simulink model "Hardware_Diagnostics_Test_backup"  (R2025b)
settings: Solver=FixedStepDiscrete  StartTime=0.0  StopTime=inf  FixedStep=0.001  RelTol=1e-3  EnableMultiTasking=on
undefined symbols (not defined in the file or in its folder): bit, Down, GPTRIP1SEL, GPTRIP2SEL, TZ1, TZ2, Up
libraries: c2802xlib x5, c280xlib x3, c2806xlib x2

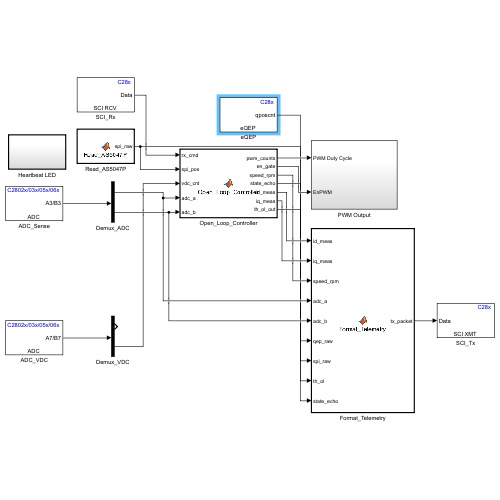
[thumbnail: Simulink's stored preview of the top-level diagram]
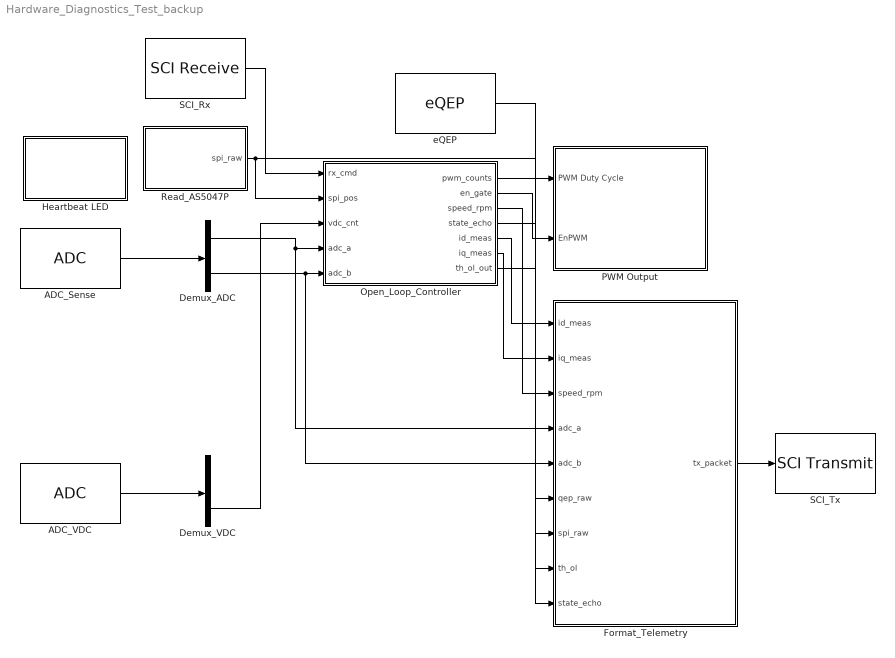
== system Hardware_Diagnostics_Test_backup ==
  ADC_Sense : c2802xlib/ADC  blkParamProc=C2000  ADCModule=1  samplingMode=Simultaneous sample mode  ADCResolution=12-bit (Single-ended input)  ADC29xResolution=12-bit  ADCMode=Single-ended input  useSOC1=SOC0  useSOC2=SOC0_SOC1  SOCAcquisitionWindow=7  SOCTriggerSource=Software  SOCInterruptTrigger=No ADCINT  Ts=-1  dType=uint16  postInterrupt=on  interruptSel=ADCINT1  ADCINTContinuous=on  endma=off  chdma=1  conv1=ADCINA0  conv2=ADCINA3 and ADCINB3  conv1_Type4=ADCIN0  conv2_Type4=ADCIN0 and ADCIN1
  ADC_VDC : c2802xlib/ADC  blkParamProc=C2000  ADCModule=1  samplingMode=Simultaneous sample mode  ADCResolution=12-bit (Single-ended input)  ADC29xResolution=12-bit  ADCMode=Single-ended input  useSOC1=SOC2  useSOC2=SOC2_SOC3  SOCAcquisitionWindow=7  SOCTriggerSource=Software  SOCInterruptTrigger=No ADCINT  Ts=-1  dType=uint16  postInterrupt=off  interruptSel=ADCINT1  ADCINTContinuous=on  endma=off  chdma=1  conv1=ADCINB7  conv2=ADCINA7 and ADCINB7  conv1_Type4=ADCIN0  conv2_Type4=ADCIN0 and ADCIN1
  Demux_ADC : Demux  Outputs=2
  Demux_VDC : Demux  Outputs=2
  Format_Telemetry : MATLAB Function  TreatAsAtomicUnit=on
  Heartbeat LED : Subsystem  TreatAsAtomicUnit=on
  Open_Loop_Controller : MATLAB Function  TreatAsAtomicUnit=on
  PWM Output : Subsystem
  Read_AS5047P : MATLAB Function  TreatAsAtomicUnit=on
  SCI_Rx : c280xlib/SCI Receive  Priority=2  sciModule=A  dataHead=''  headerCheckMaxCount=16  dataTail=''  dataType=uint8  dataLenOptions=Length via dialog  dataDim=1  maxDataLength=1  initValue=0  errOption=Output the last received value  errValue=0  sampleTime=0.001  blockingMode=off  timeOut=inf  outputStatus=off
  SCI_Tx : c280xlib/SCI Transmit  sciModule=A  dataHead='S'  dataTail='E'  frameSize=1  blockingMode=on  outputStatus=off
  eQEP : c280xlib/eQEP  useModule=eQEP1  pcInputmode=Quadrature-count  externalClockrate=2x resolution: Count the rising/falling edge  swapPolarityselection=Clockwise  qdfOutputport=off  qapPolarityselection=off  qbpPolarityselection=off  qipPolarityselection=off  qspPolarityselection=off  igatePolarityselection=off  sampleTime=0.001  pcOutputport=on  pcMaximumvalue=4095  indexInitializationcheck=off  indexInitializationevent=Falling edge  strobeInitializationcheck=off  strobeInitializationevent=Rising edge  softwareInitializationcheck=off  softwareInitializationsource=Set to init value at start up  softwareInitializationmode=on  pcInitialvalue=0  pcResetmode=Reset on the maximum position  ieloutputport=off  indexEventlatch=Rising edge  seloutputport=off  strobeEventlatch=Rising edge  pcefOutputport=off  enableEqepcapture=off  qctmrOutputport=off  qcprdOutputport=off  captureTimerprescaler=128  upEventprescaler=128  overflowErrorflag=off  directionErrorflag=off  captureTimerposition=On position counter read  unitTimerperiod=100000000  captureTimerlatch=off  capturePeriodlatch=off  positionCounterlatch=off  soenPolarityselection=off  spselPolarityselection=Index pin is used for sync output  compareValuesource=Specify via dialog  shadowMode=Load on QPOSCNT=0  compareValue=4294967295  syncOutputwidth=1  polaritySyncoutput=Active high  watchdogEnable=off  watchdogTimer=65535  outport1Datatype=auto  outport2Datatype=auto  outport3Datatype=auto  outport4Datatype=auto  outport5Datatype=auto  outport6Datatype=auto  outport7Datatype=auto  outport8Datatype=auto  outport9Datatype=auto  outport10Datatype=auto  outport11Datatype=auto  outport12Datatype=auto  eqepinterrupt_pce=off  eqepinterrupt_qpe=off  eqepinterrupt_qdc=off  eqepinterrupt_wto=off  eqepinterrupt_pcu=off  eqepinterrupt_pco=off  eqepinterrupt_pcr=off  eqepinterrupt_pcm=off  eqepinterrupt_sel=off  eqepinterrupt_iel=off  eqepinterrupt_uto=off  pheOutputport=off  watchdogOutputport=off  outport13Datatype=auto  outport14Datatype=auto
  wires:
  SCI_Rx/1 -> Open_Loop_Controller/1(rx_cmd)
  ADC_Sense/1 -> Demux_ADC/1
  Demux_ADC/2 -> Open_Loop_Controller/5(adc_b), Format_Telemetry/5(adc_b)
  Read_AS5047P/1(spi_raw) -> Open_Loop_Controller/2(spi_pos), Format_Telemetry/7(spi_raw)
  ADC_VDC/1 -> Demux_VDC/1
  Demux_ADC/1 -> Open_Loop_Controller/4(adc_a), Format_Telemetry/4(adc_a)
  Open_Loop_Controller/1(pwm_counts) -> PWM Output/1(PWM Duty Cycle)
  Open_Loop_Controller/2(en_gate) -> PWM Output/2(EnPWM)
  Format_Telemetry/1(tx_packet) -> SCI_Tx/1
  Open_Loop_Controller/5(id_meas) -> Format_Telemetry/1(id_meas)
  Open_Loop_Controller/6(iq_meas) -> Format_Telemetry/2(iq_meas)
  Open_Loop_Controller/3(speed_rpm) -> Format_Telemetry/3(speed_rpm)
  Demux_VDC/2 -> Open_Loop_Controller/3(vdc_cnt)
  eQEP/1 -> Format_Telemetry/6(qep_raw)
  Open_Loop_Controller/7(th_ol_out) -> Format_Telemetry/8(th_ol)
  Open_Loop_Controller/4(state_echo) -> Format_Telemetry/9(state_echo)

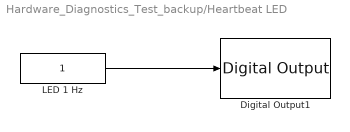
== system Hardware_Diagnostics_Test_backup/Heartbeat LED ==
  Digital Output1 : c2806xlib/Digital Output  GPIO_Number=GPIO32~GPIO39  GPIO_Bit0=off  GPIO_BIT0_Toggle=off  GPIO_Bit1=off  GPIO_BIT1_Toggle=off  GPIO_Bit2=on  GPIO_BIT2_Toggle=on  GPIO_Bit3=off  GPIO_BIT3_Toggle=off  GPIO_Bit4=off  GPIO_BIT4_Toggle=off  GPIO_Bit5=off  GPIO_BIT5_Toggle=off  GPIO_Bit6=off  GPIO_BIT6_Toggle=off  GPIO_Bit7=off  GPIO_BIT7_Toggle=off
  LED 1 Hz : Constant  OutDataTypeStr=uint16  SampleTime=0.5
  wires:
  LED 1 Hz/1 -> Digital Output1/1

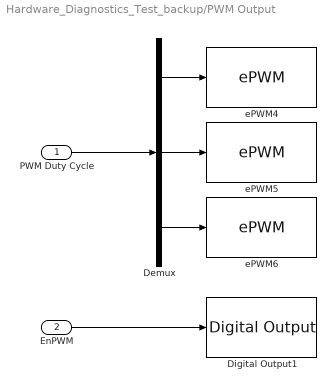
== system Hardware_Diagnostics_Test_backup/PWM Output ==
  PWM Duty Cycle : Inport
  EnPWM : Inport  Port=2
  Demux : Demux  Outputs=3
  Digital Output1 : c2806xlib/Digital Output  GPIO_Number=GPIO50~GPIO55  GPIO_Bit0=off  GPIO_BIT0_Toggle=off  GPIO_Bit1=off  GPIO_BIT1_Toggle=off  GPIO_Bit2=on  GPIO_BIT2_Toggle=off  GPIO_Bit3=off  GPIO_BIT3_Toggle=off  GPIO_Bit4=off  GPIO_BIT4_Toggle=off  GPIO_Bit5=off  GPIO_BIT5_Toggle=off  GPIO_Bit6=off  GPIO_BIT6_Toggle=off  GPIO_Bit7=off  GPIO_BIT7_Toggle=off
  ePWM4 : c2802xlib/ePWM  PwmType=C2000  useModule=ePWM4  ePWMxLINKTBPRD=Not Linked  periodUnits=Clock cycles  timerSource=Specify via dialog  timerPeriod_clk=2250  timerPeriod_sec=64000  tbshadow=Counter equals to zero  countingMode=Up-Down  phaseActiveEnable=Disable  phaseDirection=Count down after sync  phaseActive=0  synchronizationEnable=off  dcaevt1Sync=off  dcbevt1Sync=off  synchronizationOption=Counter equals to zero (CTR=Zero)  dcbevt1SyncOut=off  dcaevt1SyncOut=off  cmpdSyncOut=off  cmpcSyncOut=off  cmpbSyncOut=off  zeroSyncOut=on  swfSyncOut=off  perSynchronizationOption=Counter equals to period (CTR=PRD)  clockPrescale=1  HSclockPrescale=1  enswap=off  ePWMxAStatus=on  ePWMxAactionLogic1=Do nothing  ePWMxAactionLogic2=Do nothing  ePWMxAactionLogic3=Clear  ePWMxAactionLogic4=Set  ePWMxAactionLogic5=Do nothing  ePWMxAactionLogic6=Do nothing  ePWMxACSFenable=off  ePWMxACSFvalue=Forcing disable  ePWMxASFreload=Zero  ePWMxBStatus=off  ePWMxBactionLogic1=Do nothing  ePWMxBactionLogic2=Set  ePWMxBactionLogic3=Do nothing  ePWMxBactionLogic4=Do nothing  ePWMxBactionLogic5=Clear  ePWMxBactionLogic6=Do nothing  ePWMxBCSFenable=off  ePWMxBCSFvalue=Forcing disable  ePWMxBSFreload=Zero  ePWNxBOutWay=off  ePWMxLINKCMPA=Not Linked  CMPAUnits=Clock cycles  CMPASource=Input port  CMPAValue_per=32000  CMPAValue_clk=1125  enCMPAshadow=Counter equals to zero (CTR=Zero)  ePWMxLINKCMPB=Not Linked  CMPBUnits=Clock cycles  CMPBSource=Specify via dialog  CMPBValue_per=50  CMPBValue_clk=1125  enCMPBshadow=Counter equals to zero (CTR=Zero)  ePWMxLINKCMPC=Not Linked  CMPCUnits=Clock cycles  CMPCSource=Specify via dialog  CMPCValue_per=50  CMPCValue_clk=32000  enCMPCshadow=Counter equals to zero (CTR=Zero)  ePWMxLINKCMPD=Not Linked  CMPDUnits=Clock cycles  CMPDSource=Specify via dialog  CMPDValue_per=50  CMPDValue_clk=32000  enCMPDshadow=Counter equals to zero (CTR=Zero)  enableDBePWMxA=on  enableDBePWMxB=on  enhalfcycle=off  DBpolarity=Active high complementary (AHC)  DBedgeDelay=Positive  DBSource_ePWMxA=ePWMxA  DBSource_ePWMxB=ePWMxA  DBPeriodUnits=Clock cycles  DBperiodSource=Specify via dialog  REDperiod=5  FEDperiod=5  REDperiod_sec=0  FEDperiod_sec=0  LoadModeDBRED=Immediate without using shadow  LoadModeDBFED=Immediate without using shadow  adcstartModuleA=on  adcrequestEventA=First event  adcstartEventA=Counter equals to period (CTR=PRD)  adcstartEventA_type2=Digital Compare Module A Event 1 start of conversion (DCAEVT1.soc)  adcstartModuleB=off  adcrequestEventB=First event  adcstartEventB=Counter equals to zero (CTR=Zero)  adcstartEventB_type2=Counter equals to zero (CTR=Zero)  intEn=off  intPrd=First event  intSel=Counter equals to zero (CTR=Zero)  intSel_type2=Counter equals to zero (CTR=Zero)  hrpe=off  enHRPWM=off  HRPWM_LoadMode=Counter equals to period (CTR=PRD)  HRPWM_CTLMode=Duty or Period control mode  HRPWM_EDGMode=Both edge  hrpeb=off  enHRPWMB=off  HRPWM_LoadModeB=Counter equals to zero (CTR=ZERO)  HRPWM_CTLModeB=Duty or Period control mode  HRPWM_EDGModeB=Both edge  enHRDBRED=off  enHRDBFED=off  enSFO=on  enautoconv=on  chopperEnable=off  chopperFrequency=1  chopperFirstwidth=1  chopperDuty=12.5%  tripZonesource=Specify via dialog  tzselOSHT1=off  tzselOSHT2=off  tzselOSHT3=off  tzselOSHT4=off  tzselOSHT5=off  tzselOSHT6=off  tzselOSHDCAEV1=off  tzselOSHDCBEV1=off  tzselCBC1=off  tzselCBC2=off  tzselCBC3=off  tzselCBC4=off  tzselCBC5=off  tzselCBC6=off  tzselCBCDCAEV2=off  tzselCBCDCBEV2=off  enTzOstIntr=off  enTzCbcIntr=off  enTzDCAEVT1Intr=off  enTzDCAEVT2Intr=off  enTzDCBEVT1Intr=off  enTzDCBEVT2Intr=off  tzclrCBCLatch=Counter equals to zero (CTR=Zero)  ePWMxAforced=No action  ePWMxBforced=No action  DCAEVT1forced=No action  DCBEVT1forced=No action  DCAEVT2forced=No action  DCBEVT2forced=No action  dcah=Trip Zone 1 input (TZ1)  dcal=Trip Zone 2 input (TZ2)  dcbh=Trip Zone 1 input (TZ1)  dcbl=Trip Zone 2 input (TZ2)  dcah_type2=GPTRIP1SEL/(TZ1)  dcal_type2=GPTRIP2SEL/(TZ2)  dcbh_type2=GPTRIP1SEL/(TZ1)  dcbl_type2=GPTRIP2SEL/(TZ2)  gendcaevt1=Event disabled  gendcaevt2=Event disabled  gendcbevt1=Event disabled  gendcbevt2=Event disabled  dcaevt1src=DCAEVT1 with sync  dcaevt2src=DCAEVT2 with sync  dcbevt1src=DCBEVT1 with sync  dcbevt2src=DCBEVT2 with sync  pulsesel=Counter equals to zero (CTR=Zero)  blankinv=off  blankoffset=0  blankwidth=0  evsrcsel=Filtered version of DCAEVT1 (DCAEVT1FILT)  encape=off
  ePWM5 : c2802xlib/ePWM  PwmType=C2000  useModule=ePWM5  ePWMxLINKTBPRD=Not Linked  periodUnits=Clock cycles  timerSource=Specify via dialog  timerPeriod_clk=2250  timerPeriod_sec=64000  tbshadow=Counter equals to zero  countingMode=Up-Down  phaseActiveEnable=Set counter to phase value specified via dialog  phaseDirection=Count up after sync  phaseActive=0  synchronizationEnable=off  dcaevt1Sync=off  dcbevt1Sync=off  synchronizationOption=Pass through (EPWMxSYNCI or SWFSYNC)  dcbevt1SyncOut=off  dcaevt1SyncOut=off  cmpdSyncOut=off  cmpcSyncOut=off  cmpbSyncOut=off  zeroSyncOut=off  swfSyncOut=on  perSynchronizationOption=Counter equals to period (CTR=PRD)  clockPrescale=1  HSclockPrescale=1  enswap=off  ePWMxAStatus=on  ePWMxAactionLogic1=Do nothing  ePWMxAactionLogic2=Do nothing  ePWMxAactionLogic3=Clear  ePWMxAactionLogic4=Set  ePWMxAactionLogic5=Do nothing  ePWMxAactionLogic6=Do nothing  ePWMxACSFenable=off  ePWMxACSFvalue=Forcing disable  ePWMxASFreload=Zero  ePWMxBStatus=off  ePWMxBactionLogic1=Do nothing  ePWMxBactionLogic2=Set  ePWMxBactionLogic3=Do nothing  ePWMxBactionLogic4=Do nothing  ePWMxBactionLogic5=Clear  ePWMxBactionLogic6=Do nothing  ePWMxBCSFenable=off  ePWMxBCSFvalue=Forcing disable  ePWMxBSFreload=Zero  ePWNxBOutWay=off  ePWMxLINKCMPA=Not Linked  CMPAUnits=Clock cycles  CMPASource=Input port  CMPAValue_per=32000  CMPAValue_clk=1125  enCMPAshadow=Counter equals to zero (CTR=Zero)  ePWMxLINKCMPB=Not Linked  CMPBUnits=Clock cycles  CMPBSource=Specify via dialog  CMPBValue_per=50  CMPBValue_clk=1125  enCMPBshadow=Counter equals to zero (CTR=Zero)  ePWMxLINKCMPC=Not Linked  CMPCUnits=Clock cycles  CMPCSource=Specify via dialog  CMPCValue_per=50  CMPCValue_clk=32000  enCMPCshadow=Counter equals to zero (CTR=Zero)  ePWMxLINKCMPD=Not Linked  CMPDUnits=Clock cycles  CMPDSource=Specify via dialog  CMPDValue_per=50  CMPDValue_clk=32000  enCMPDshadow=Counter equals to zero (CTR=Zero)  enableDBePWMxA=on  enableDBePWMxB=on  enhalfcycle=off  DBpolarity=Active high complementary (AHC)  DBedgeDelay=Positive  DBSource_ePWMxA=ePWMxA  DBSource_ePWMxB=ePWMxA  DBPeriodUnits=Clock cycles  DBperiodSource=Specify via dialog  REDperiod=5  FEDperiod=5  REDperiod_sec=0  FEDperiod_sec=0  LoadModeDBRED=Immediate without using shadow  LoadModeDBFED=Immediate without using shadow  adcstartModuleA=off  adcrequestEventA=First event  adcstartEventA=Digital Compare Module A Event 1 start of conversion (DCAEVT1.soc)  adcstartEventA_type2=Digital Compare Module A Event 1 start of conversion (DCAEVT1.soc)  adcstartModuleB=off  adcrequestEventB=First event  adcstartEventB=Counter equals to zero (CTR=Zero)  adcstartEventB_type2=Counter equals to zero (CTR=Zero)  intEn=off  intPrd=First event  intSel=Counter equals to zero (CTR=Zero)  intSel_type2=Counter equals to zero (CTR=Zero)  hrpe=off  enHRPWM=off  HRPWM_LoadMode=Counter equals to period (CTR=PRD)  HRPWM_CTLMode=Duty or Period control mode  HRPWM_EDGMode=Both edge  hrpeb=off  enHRPWMB=off  HRPWM_LoadModeB=Counter equals to zero (CTR=ZERO)  HRPWM_CTLModeB=Duty or Period control mode  HRPWM_EDGModeB=Both edge  enHRDBRED=off  enHRDBFED=off  enSFO=on  enautoconv=on  chopperEnable=off  chopperFrequency=1  chopperFirstwidth=1  chopperDuty=12.5%  tripZonesource=Specify via dialog  tzselOSHT1=off  tzselOSHT2=off  tzselOSHT3=off  tzselOSHT4=off  tzselOSHT5=off  tzselOSHT6=off  tzselOSHDCAEV1=off  tzselOSHDCBEV1=off  tzselCBC1=off  tzselCBC2=off  tzselCBC3=off  tzselCBC4=off  tzselCBC5=off  tzselCBC6=off  tzselCBCDCAEV2=off  tzselCBCDCBEV2=off  enTzOstIntr=off  enTzCbcIntr=off  enTzDCAEVT1Intr=off  enTzDCAEVT2Intr=off  enTzDCBEVT1Intr=off  enTzDCBEVT2Intr=off  tzclrCBCLatch=Counter equals to zero (CTR=Zero)  ePWMxAforced=No action  ePWMxBforced=No action  DCAEVT1forced=No action  DCBEVT1forced=No action  DCAEVT2forced=No action  DCBEVT2forced=No action  dcah=Trip Zone 1 input (TZ1)  dcal=Trip Zone 2 input (TZ2)  dcbh=Trip Zone 1 input (TZ1)  dcbl=Trip Zone 2 input (TZ2)  dcah_type2=GPTRIP1SEL/(TZ1)  dcal_type2=GPTRIP2SEL/(TZ2)  dcbh_type2=GPTRIP1SEL/(TZ1)  dcbl_type2=GPTRIP2SEL/(TZ2)  gendcaevt1=Event disabled  gendcaevt2=Event disabled  gendcbevt1=Event disabled  gendcbevt2=Event disabled  dcaevt1src=DCAEVT1 with sync  dcaevt2src=DCAEVT2 with sync  dcbevt1src=DCBEVT1 with sync  dcbevt2src=DCBEVT2 with sync  pulsesel=Counter equals to zero (CTR=Zero)  blankinv=off  blankoffset=0  blankwidth=0  evsrcsel=Filtered version of DCAEVT1 (DCAEVT1FILT)  encape=off
  ePWM6 : c2802xlib/ePWM  PwmType=C2000  useModule=ePWM6  ePWMxLINKTBPRD=Not Linked  periodUnits=Clock cycles  timerSource=Specify via dialog  timerPeriod_clk=2250  timerPeriod_sec=64000  tbshadow=Counter equals to zero  countingMode=Up-Down  phaseActiveEnable=Set counter to phase value specified via dialog  phaseDirection=Count up after sync  phaseActive=0  synchronizationEnable=off  dcaevt1Sync=off  dcbevt1Sync=off  synchronizationOption=Disable  dcbevt1SyncOut=off  dcaevt1SyncOut=off  cmpdSyncOut=off  cmpcSyncOut=off  cmpbSyncOut=off  zeroSyncOut=off  swfSyncOut=off  perSynchronizationOption=Counter equals to period (CTR=PRD)  clockPrescale=1  HSclockPrescale=1  enswap=off  ePWMxAStatus=on  ePWMxAactionLogic1=Do nothing  ePWMxAactionLogic2=Do nothing  ePWMxAactionLogic3=Clear  ePWMxAactionLogic4=Set  ePWMxAactionLogic5=Do nothing  ePWMxAactionLogic6=Do nothing  ePWMxACSFenable=off  ePWMxACSFvalue=Forcing disable  ePWMxASFreload=Zero  ePWMxBStatus=off  ePWMxBactionLogic1=Do nothing  ePWMxBactionLogic2=Set  ePWMxBactionLogic3=Do nothing  ePWMxBactionLogic4=Do nothing  ePWMxBactionLogic5=Clear  ePWMxBactionLogic6=Do nothing  ePWMxBCSFenable=off  ePWMxBCSFvalue=Forcing disable  ePWMxBSFreload=Zero  ePWNxBOutWay=off  ePWMxLINKCMPA=Not Linked  CMPAUnits=Clock cycles  CMPASource=Input port  CMPAValue_per=32000  CMPAValue_clk=1125  enCMPAshadow=Counter equals to zero (CTR=Zero)  ePWMxLINKCMPB=Not Linked  CMPBUnits=Clock cycles  CMPBSource=Specify via dialog  CMPBValue_per=50  CMPBValue_clk=1125  enCMPBshadow=Counter equals to zero (CTR=Zero)  ePWMxLINKCMPC=Not Linked  CMPCUnits=Clock cycles  CMPCSource=Specify via dialog  CMPCValue_per=50  CMPCValue_clk=32000  enCMPCshadow=Counter equals to zero (CTR=Zero)  ePWMxLINKCMPD=Not Linked  CMPDUnits=Clock cycles  CMPDSource=Specify via dialog  CMPDValue_per=50  CMPDValue_clk=32000  enCMPDshadow=Counter equals to zero (CTR=Zero)  enableDBePWMxA=on  enableDBePWMxB=on  enhalfcycle=off  DBpolarity=Active high complementary (AHC)  DBedgeDelay=Positive  DBSource_ePWMxA=ePWMxA  DBSource_ePWMxB=ePWMxA  DBPeriodUnits=Clock cycles  DBperiodSource=Specify via dialog  REDperiod=5  FEDperiod=5  REDperiod_sec=0  FEDperiod_sec=0  LoadModeDBRED=Immediate without using shadow  LoadModeDBFED=Immediate without using shadow  adcstartModuleA=off  adcrequestEventA=First event  adcstartEventA=Digital Compare Module A Event 1 start of conversion (DCAEVT1.soc)  adcstartEventA_type2=Digital Compare Module A Event 1 start of conversion (DCAEVT1.soc)  adcstartModuleB=off  adcrequestEventB=First event  adcstartEventB=Counter equals to zero (CTR=Zero)  adcstartEventB_type2=Counter equals to zero (CTR=Zero)  intEn=off  intPrd=First event  intSel=Counter equals to zero (CTR=Zero)  intSel_type2=Counter equals to zero (CTR=Zero)  hrpe=off  enHRPWM=off  HRPWM_LoadMode=Counter equals to period (CTR=PRD)  HRPWM_CTLMode=Duty or Period control mode  HRPWM_EDGMode=Both edge  hrpeb=off  enHRPWMB=off  HRPWM_LoadModeB=Counter equals to zero (CTR=ZERO)  HRPWM_CTLModeB=Duty or Period control mode  HRPWM_EDGModeB=Both edge  enHRDBRED=off  enHRDBFED=off  enSFO=on  enautoconv=on  chopperEnable=off  chopperFrequency=1  chopperFirstwidth=1  chopperDuty=12.5%  tripZonesource=Specify via dialog  tzselOSHT1=off  tzselOSHT2=off  tzselOSHT3=off  tzselOSHT4=off  tzselOSHT5=off  tzselOSHT6=off  tzselOSHDCAEV1=off  tzselOSHDCBEV1=off  tzselCBC1=off  tzselCBC2=off  tzselCBC3=off  tzselCBC4=off  tzselCBC5=off  tzselCBC6=off  tzselCBCDCAEV2=off  tzselCBCDCBEV2=off  enTzOstIntr=off  enTzCbcIntr=off  enTzDCAEVT1Intr=off  enTzDCAEVT2Intr=off  enTzDCBEVT1Intr=off  enTzDCBEVT2Intr=off  tzclrCBCLatch=Counter equals to zero (CTR=Zero)  ePWMxAforced=No action  ePWMxBforced=No action  DCAEVT1forced=No action  DCBEVT1forced=No action  DCAEVT2forced=No action  DCBEVT2forced=No action  dcah=Trip Zone 1 input (TZ1)  dcal=Trip Zone 2 input (TZ2)  dcbh=Trip Zone 1 input (TZ1)  dcbl=Trip Zone 2 input (TZ2)  dcah_type2=GPTRIP1SEL/(TZ1)  dcal_type2=GPTRIP2SEL/(TZ2)  dcbh_type2=GPTRIP1SEL/(TZ1)  dcbl_type2=GPTRIP2SEL/(TZ2)  gendcaevt1=Event disabled  gendcaevt2=Event disabled  gendcbevt1=Event disabled  gendcbevt2=Event disabled  dcaevt1src=DCAEVT1 with sync  dcaevt2src=DCAEVT2 with sync  dcbevt1src=DCBEVT1 with sync  dcbevt2src=DCBEVT2 with sync  pulsesel=Counter equals to zero (CTR=Zero)  blankinv=off  blankoffset=0  blankwidth=0  evsrcsel=Filtered version of DCAEVT1 (DCAEVT1FILT)  encape=off
  wires:
  Demux/1 -> ePWM4/1
  Demux/2 -> ePWM5/1
  PWM Duty Cycle/1 -> Demux/1
  Demux/3 -> ePWM6/1
  EnPWM/1 -> Digital Output1/1

== matlab function Hardware_Diagnostics_Test_backup/Read_AS5047P ==
function spi_raw = Read_AS5047P()
%#codegen
persistent init_done
spi_raw = uint16(0);
if coder.target('Rtw')
    coder.cinclude('as5047p_spi.h');
    coder.updateBuildInfo('addSourceFiles', 'as5047p_spi.c');
    coder.updateBuildInfo('addIncludePaths', 'c:\96v_gan_humanoid_drive\phase1\simulation\MyFOC code');
    if isempty(init_done)
        coder.ceval('as5047p_spi_init');
        init_done = true;
    end
    coder.ceval('as5047p_spi_read', coder.ref(spi_raw));
end

== matlab function Hardware_Diagnostics_Test_backup/Format_Telemetry ==
function tx_packet = Format_Telemetry(id_meas, iq_meas, speed_rpm, adc_a, adc_b, qep_raw, spi_raw, th_ol, state_echo)
%#codegen
    tx_packet = zeros(19, 1, 'uint8');
    id_i16 = int16(round(id_meas * single(100.0)));
    iq_i16 = int16(round(iq_meas * single(100.0)));
    id_u16 = typecast(id_i16, 'uint16');
    iq_u16 = typecast(iq_i16, 'uint16');
    spd_u16 = typecast(int16(round(speed_rpm)), 'uint16');
    aa = uint16(adc_a);
    ab = uint16(adc_b);
    qep_val = uint16(qep_raw);
    spi_val = uint16(spi_raw);
    % Normalize th_ol (0 to 2*pi) to uint16 (0 to 65535)
    th_norm = th_ol * single(10430.37835); % 65535 / (2*pi)
    if th_norm < single(0.0), th_norm = single(0.0); end
    if th_norm > single(65535.0), th_norm = single(65535.0); end
    th_u16 = uint16(th_norm);
    echo = uint8(state_echo);

    tx_packet(1) = uint8(170);
    tx_packet(2) = uint8(85);
    % High byte first (Big-Endian)
    tx_packet(3) = uint8(bitshift(id_u16, -8));
    tx_packet(4) = uint8(bitand(id_u16, 255));
    tx_packet(5) = uint8(bitshift(iq_u16, -8));
    tx_packet(6) = uint8(bitand(iq_u16, 255));
    tx_packet(7) = uint8(bitshift(spd_u16, -8));
    tx_packet(8) = uint8(bitand(spd_u16, 255));
    tx_packet(9) = uint8(bitshift(aa, -8));
    tx_packet(10) = uint8(bitand(aa, 255));
    tx_packet(11) = uint8(bitshift(ab, -8));
    tx_packet(12) = uint8(bitand(ab, 255));
    tx_packet(13) = uint8(bitshift(spi_val, -8));
    tx_packet(14) = uint8(bitand(spi_val, 255));
    tx_packet(15) = uint8(bitshift(qep_val, -8));
    tx_packet(16) = uint8(bitand(qep_val, 255));
    tx_packet(17) = uint8(bitshift(th_u16, -8));
    tx_packet(18) = uint8(bitand(th_u16, 255));
    tx_packet(19) = echo;
end

== matlab function Hardware_Diagnostics_Test_backup/Open_Loop_Controller ==
function [pwm_counts, en_gate, speed_rpm, state_echo, id_meas, iq_meas, th_ol_out] = Open_Loop_Controller(rx_cmd, spi_pos, vdc_cnt, adc_a, adc_b)
%#codegen
    % Preallocate outputs
    pwm_counts = single([1125.0; 1125.0; 1125.0]);
    en_gate = false;
    speed_rpm = single(0.0);
    state_echo = uint8(0);
    id_meas = single(0.0);
    iq_meas = single(0.0);
    th_ol_out = single(0.0);

    persistent state theta_ol last_spi_pos filt_speed th_align align_done align_timer ...
               spd_int id_int iq_int
    if isempty(state)
        state = uint8(0);
        theta_ol = single(0.0);
        last_spi_pos = uint16(0);
        filt_speed = single(0.0);
        th_align = single(5.4437); % Default 311.9 deg
        align_done = false;
        align_timer = uint16(0);
        spd_int = single(0.0);
        id_int  = single(0.0);
        iq_int  = single(0.0);
    end

    % Constants
    TWO_PI = single(6.283185307);
    TWO_PI_OVER_3 = single(2.094395102);
    POLE_PAIRS = single(21.0);
    ONE_OVER_SQRT3 = single(0.577350269);
    SQRT3_OVER_2   = single(0.866025404);

    % 1. Vdc Calculation
    vdc_raw_volts = single(vdc_cnt) * single(3.3 * 46.4545 / 4095.0);
    if vdc_raw_volts > single(10.0)
        offset_a = single(2041.0);
        offset_b = single(2059.0);
        vdc_volts = vdc_raw_volts;
    else
        offset_a = single(2041.0);
        offset_b = single(2059.0);
        vdc_volts = single(40.0);
    end

    % 2. Speed Calculation from AS5047P SPI
    cur_pos = int32(spi_pos);
    prev_pos = int32(last_spi_pos);
    delta_pos = cur_pos - prev_pos;
    if delta_pos > 8192
        delta_pos = delta_pos - 16384;
    elseif delta_pos < -8192
        delta_pos = delta_pos + 16384;
    end
    last_spi_pos = uint16(spi_pos);
    raw_rpm = single(delta_pos) * single(3.662109375);
    filt_speed = single(0.85) * filt_speed + single(0.15) * raw_rpm;
    speed_rpm = filt_speed;

    % 3. Mechanical & Electrical Angle from AS5047P Absolute SPI
    th_m = (single(spi_pos) / single(16384.0)) * TWO_PI;
    th_e_unmod = POLE_PAIRS * (th_m - th_align);
    th_e = mod(th_e_unmod, TWO_PI);
    if th_e < single(0.0)
        th_e = th_e + TWO_PI;
    end

    % 4. Current Measurement & Transforms (Clarke & Park)
    I_SCALE = single(0.02014652); % (3.3/4095)/(0.002*20)
    ia = (single(adc_a) - offset_a) * I_SCALE;
    ib = (single(adc_b) - offset_b) * I_SCALE;
    i_alpha = ia;
    i_beta  = (ia + single(2.0) * ib) * ONE_OVER_SQRT3;

    cos_e = cos(th_e);
    sin_e = sin(th_e);
    id_meas =  i_alpha * cos_e + i_beta * sin_e;
    iq_meas = -i_alpha * sin_e + i_beta * cos_e;

    % 5. Automatic Startup Alignment (When Vdc > 30V on boot)
    if ~align_done && vdc_volts >= single(30.0)
        align_timer = align_timer + uint16(1);
        m_align = single(0.04); % Safe 4% modulation at 40V = 1.6V (~3.6A peak during pull-in)
        da = single(0.5) + m_align;
        db = single(0.5) - m_align * single(0.5);
        dc = single(0.5) - m_align * single(0.5);
        pwm_counts = [da * single(2250.0); db * single(2250.0); dc * single(2250.0)];
        en_gate = true;
        state_echo = uint8(9); % State 9 = AUTO-ALIGNING
        if align_timer >= uint16(1500) % 1.5 seconds settling
            th_align = th_m;           % Latch absolute mechanical angle at 0 deg elec
            align_done = true;
            state = uint8(0);          % Enter Idle/Stopped
            en_gate = false;
        end
        th_ol_out = single(0.0);
        return;
    end

    % 6. Command Decoding
    last_state = state;
    if rx_cmd == uint8('0') || rx_cmd == uint8(48) || rx_cmd == uint8('s') || rx_cmd == uint8('S')
        state = uint8(0);
    elseif rx_cmd == uint8(1) || rx_cmd == uint8('1') || rx_cmd == uint8('r') || rx_cmd == uint8('R')
        state = uint8(1);
    elseif rx_cmd == uint8(2) || rx_cmd == uint8('2')
        state = uint8(2);
    elseif rx_cmd == uint8(3) || rx_cmd == uint8('3')
        state = uint8(3);
    elseif rx_cmd == uint8(4) || rx_cmd == uint8('4') || rx_cmd == uint8('a') || rx_cmd == uint8('A')
        state = uint8(4);
    elseif rx_cmd == uint8(5) || rx_cmd == uint8('5')
        state = uint8(5); % Closed-Loop FOC 100 RPM
    elseif rx_cmd == uint8(6) || rx_cmd == uint8('6')
        state = uint8(6); % Closed-Loop FOC 200 RPM
    elseif rx_cmd == uint8(7) || rx_cmd == uint8('7')
        state = uint8(7); % Closed-Loop FOC -100 RPM
    end

    if state ~= last_state
        spd_int = single(0.0);
        id_int  = single(0.0);
        iq_int  = single(0.0);
    end

    % 7. Mode Execution
    if state == uint8(0)
        % IDLE / STOPPED
        pwm_counts = single([1125.0; 1125.0; 1125.0]);
        en_gate = false;
        spd_int = single(0.0);
        id_int  = single(0.0);
        iq_int  = single(0.0);
        state_echo = uint8(0);

    elseif state == uint8(1) || state == uint8(2) || state == uint8(3)
        % Open Loop Mode
        if state == uint8(1)
            w_e = single(50.26548); % 60 RPM
        elseif state == uint8(2)
            w_e = single(100.53096); % 120 RPM
        else
            w_e = single(-50.26548); % -60 RPM
        end
        theta_ol = theta_ol + w_e * single(0.001);
        if theta_ol >= TWO_PI
            theta_ol = theta_ol - TWO_PI;
        elseif theta_ol < single(0.0)
            theta_ol = theta_ol + TWO_PI;
        end
        m_ol = single(0.06);
        da = single(0.5) + m_ol * cos(theta_ol);
        db = single(0.5) + m_ol * cos(theta_ol - TWO_PI_OVER_3);
        dc = single(0.5) + m_ol * cos(theta_ol + TWO_PI_OVER_3);
        pwm_counts = [da * single(2250.0); db * single(2250.0); dc * single(2250.0)];
        en_gate = true;
        state_echo = state;

    elseif state == uint8(4)
        % Manual Alignment Mode (0 deg Elec)
        m_align = single(0.04);
        da = single(0.5) + m_align;
        db = single(0.5) - m_align * single(0.5);
        dc = single(0.5) - m_align * single(0.5);
        pwm_counts = [da * single(2250.0); db * single(2250.0); dc * single(2250.0)];
        en_gate = true;
        th_align = th_m;
        align_done = true;
        state_echo = uint8(4);

    else
        % TRUE CLOSED-LOOP FOC (Dual PI Current Loops + Outer Speed Loop)
        if state == uint8(5)
            w_target = single(100.0); % +100 RPM
        elseif state == uint8(6)
            w_target = single(200.0); % +200 RPM
        else
            w_target = single(-100.0); % -100 RPM
        end

        % Outer Speed PI Loop -> Iq_target
        err_w = w_target - speed_rpm;
        KP_SPD = single(0.025);   % 0.025 A / RPM
        KI_SPD = single(0.040);   % 0.040 A / (RPM * s)
        I_MAX_SAFE = single(2.5); % Hard-limit current to 2.5 A (prevents bench supply trips!)

        spd_int = spd_int + KI_SPD * single(0.001) * err_w;
        if spd_int > I_MAX_SAFE,  spd_int = I_MAX_SAFE;  end
        if spd_int < -I_MAX_SAFE, spd_int = -I_MAX_SAFE; end

        iq_ref = KP_SPD * err_w + spd_int;
        if iq_ref > I_MAX_SAFE,  iq_ref = I_MAX_SAFE;  end
        if iq_ref < -I_MAX_SAFE, iq_ref = -I_MAX_SAFE; end
        id_ref = single(0.0); % Pure torque mode (Id = 0)

        % Inner Current PI Regulators (Id and Iq)
        err_id = id_ref - id_meas;
        err_iq = iq_ref - iq_meas;
        KP_CURR = single(0.25);   % V / A
        KI_CURR = single(0.20);   % V / A per ms step
        V_MAX_LINEAR = single(0.577) * vdc_volts; % Max SVPWM linear voltage (~23V at 40V)

        % Id PI controller
        id_int = id_int + KI_CURR * err_id;
        if id_int > V_MAX_LINEAR,  id_int = V_MAX_LINEAR;  end
        if id_int < -V_MAX_LINEAR, id_int = -V_MAX_LINEAR; end
        vd_cmd = KP_CURR * err_id + id_int;

        % Iq PI controller + Back-EMF Feedforward
        bemf_ff = speed_rpm * single(0.033); % Ke = 33 V/krpm = 0.033 V/RPM
        iq_int = iq_int + KI_CURR * err_iq;
        if iq_int > V_MAX_LINEAR,  iq_int = V_MAX_LINEAR;  end
        if iq_int < -V_MAX_LINEAR, iq_int = -V_MAX_LINEAR; end
        vq_cmd = KP_CURR * err_iq + iq_int + bemf_ff;

        % Voltage Vector Saturation
        v_mag = sqrt(vd_cmd * vd_cmd + vq_cmd * vq_cmd);
        if v_mag > V_MAX_LINEAR
            v_scale = V_MAX_LINEAR / v_mag;
            vd_cmd = vd_cmd * v_scale;
            vq_cmd = vq_cmd * v_scale;
        end

        % Inverse Park Transform
        v_alpha = vd_cmd * cos_e - vq_cmd * sin_e;
        v_beta  = vd_cmd * sin_e + vq_cmd * cos_e;

        % Inverse Clarke Transform
        va = v_alpha;
        vb = single(-0.5) * v_alpha + SQRT3_OVER_2 * v_beta;
        vc = single(-0.5) * v_alpha - SQRT3_OVER_2 * v_beta;

        % Space Vector Neutral-Point Modulation (Center-aligned)
        v_min = min(min(va, vb), vc);
        v_max = max(max(va, vb), vc);
        v_com = single(0.5) * (v_min + v_max);
        da = single(0.5) + (va - v_com) / vdc_volts;
        db = single(0.5) + (vb - v_com) / vdc_volts;
        dc = single(0.5) + (vc - v_com) / vdc_volts;

        % Duty Cycle Clamping (2% to 98%)
        if da < single(0.02), da = single(0.02); elseif da > single(0.98), da = single(0.98); end
        if db < single(0.02), db = single(0.02); elseif db > single(0.98), db = single(0.98); end
        if dc < single(0.02), dc = single(0.02); elseif dc > single(0.98), dc = single(0.98); end

        pwm_counts = [da * single(2250.0); db * single(2250.0); dc * single(2250.0)];
        en_gate = true;
        state_echo = state;
    end
    th_ol_out = theta_ol;
end
